simulink model "project2_model"  (R2014a)
settings: Solver=ode45  StartTime=0.0  StopTime=2  RelTol=1e-3
InitFcn:
  | G32I = [-1 -1 -1 1  1 1 -1 -1   1 1 1 1  1 -1 -1 -1   -1 1 -1 1   1 -1 -1 -1   1 1 -1 -1  -1 1 -1 1];
  | 
  | G32IR = [1 -1 1 -1 -1 -1 1 1 -1 -1 -1 1 1 -1 1 -1 -1 -1 -1 1 1 1 1 1 -1 -1 1 1  1 -1 -1 -1 ];
  | 
  | G32Q = [ 1 1 -1 1    -1 1 1 1   1 -1 1 -1   -1 1 -1 1    1 -1 1 -1   1 -1 -1 -1   -1 1 -1 1   -1 1 -1 -1  ];
  | 
  | G32QR = [ -1 -1 1 -1   1 -1 1 -1   -1 -1 -1 1   -1 1 -1 1   1 -1 1 -1   -1 1 -1 1   1  1 1 -1   1 -1 1 1 ];
libraries: simulink x3, simulink_extras x2, dspindex x2, dspsigops x1
settings Model: Creator=JohnE  LastModifiedBy=kastner

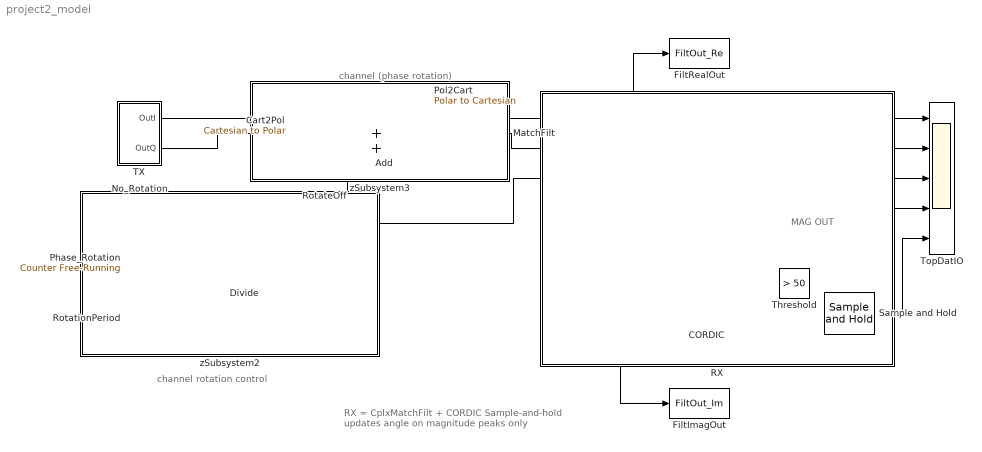
== system project2_model ==
  note: RX = CplxMatchFilt + CORDIC
      | Sample-and-hold updates angle on magnitude
      | peaks only
  note: MAG OUT
  note: channel rotation control
  note: channel (phase rotation)
  Add : Sum
  CORDIC : Subsystem
  Cart2Pol : simulink_extras/Transformations/Cartesian to Polar
  Divide : Product  Inputs=*/
  FiltImagOut : ToWorkspace  VariableName=FiltOut_Im  SaveFormat=Structure  SampleTime=-1
  FiltRealOut : ToWorkspace  VariableName=FiltOut_Re  SaveFormat=Structure  SampleTime=-1
  MatchFilt : Subsystem
  No_Rotation : Constant  Value=0
  Phase_Rotation : simulink/Sources/Counter Free-Running  NumBits=16  tsamp=-1
  Pol2Cart : simulink_extras/Transformations/Polar to Cartesian
  RX : Subsystem
      mask Display: disp('');
  RotateOff : ManualSwitch  CurrentSetting=0
  RotationPeriod : Constant  Value=1000
  Sample and Hold : dspsigops/Sample and Hold  trig=Rising edge  initCond=0  latchinput=off
  TX : Subsystem
  Threshold : simulink/Logic and Bit Operations/Compare To Constant  relop=>  const=50  OutDataTypeStr=boolean
  TopDatIO : Scope  NumInputPorts=5
      settings: YMin=-2.2~30.4~30~30.4~-5  YMax=2.2~33.6~42.5~33.6~5  SaveName=ScopeData5  MaxDataPoints=220000
  zSubsystem2 : Subsystem
      mask Display: disp('');
  zSubsystem3 : Subsystem
      mask Display: disp('');
  wires:
  MatchFilt/1(OutRe) -> CORDIC/1(XIn), TopDatIO/1, FiltRealOut/1
  MatchFilt/2(OutIm) -> FiltImagOut/1, CORDIC/2(YIn), TopDatIO/2
  TX/1(OutI) -> Cart2Pol/1
  TX/2(OutQ) -> Cart2Pol/2
  Cart2Pol/1 -> Pol2Cart/1
  Pol2Cart/1 -> MatchFilt/1(InI)
  Pol2Cart/2 -> MatchFilt/2(InQ)
  Cart2Pol/2 -> Add/1
  Add/1 -> Pol2Cart/2
  Phase_Rotation/1 -> Divide/1
  Divide/1 -> RotateOff/2
  RotationPeriod/1 -> Divide/2
  Sample and Hold/1 -> TopDatIO/5
  Threshold/1 -> Sample and Hold/Trigger
  RotateOff/1 -> Add/2, TopDatIO/3
  No_Rotation/1 -> RotateOff/1
  CORDIC/1(Mag) -> TopDatIO/4, Threshold/1
  CORDIC/2(Angle) -> Sample and Hold/1

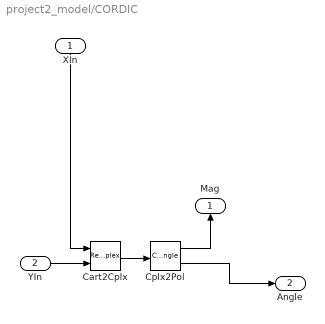
== system project2_model/CORDIC ==
  XIn : Inport
  YIn : Inport  Port=2
  Cart2Cplx : RealImagToComplex
  Cplx2Pol : ComplexToMagnitudeAngle
  Mag : Outport
  Angle : Outport  Port=2
  wires:
  XIn/1 -> Cart2Cplx/1
  YIn/1 -> Cart2Cplx/2
  Cplx2Pol/1 -> Mag/1
  Cart2Cplx/1 -> Cplx2Pol/1
  Cplx2Pol/2 -> Angle/1

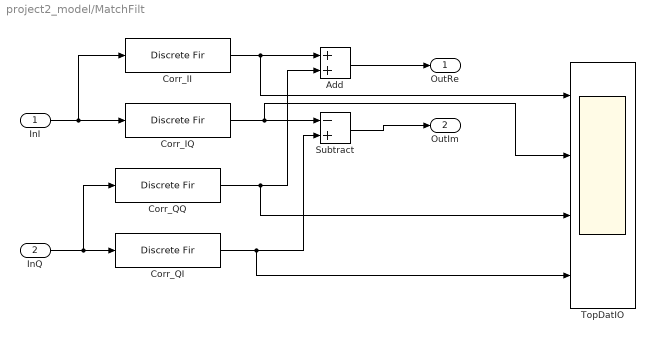
== system project2_model/MatchFilt ==
  InI : Inport
  InQ : Inport  Port=2
  Add : Sum
  Corr_II : DiscreteFir  Coefficients=G32IR
  Corr_IQ : DiscreteFir  Coefficients=G32QR
  Corr_QI : DiscreteFir  Coefficients=G32IR
  Corr_QQ : DiscreteFir  Coefficients=G32QR
  Subtract : Sum  Inputs=-+
  TopDatIO : Scope  NumInputPorts=4
      settings: YMin=-2.2~30.4~30~30.4  YMax=2.2~33.6~42.5~33.6  MaxDataPoints=220000
  OutRe : Outport
  OutIm : Outport  Port=2
  wires:
  InQ/1 -> Corr_QQ/1, Corr_QI/1
  InI/1 -> Corr_II/1, Corr_IQ/1
  Add/1 -> OutRe/1
  Corr_QQ/1 -> TopDatIO/3, Add/2
  Corr_QI/1 -> TopDatIO/4, Subtract/2
  Subtract/1 -> OutIm/1
  Corr_IQ/1 -> TopDatIO/2, Subtract/1
  Corr_II/1 -> TopDatIO/1, Add/1

== system project2_model/RX ==

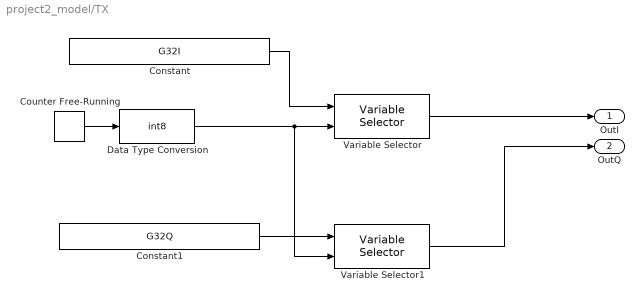
== system project2_model/TX ==
  Constant : Constant  Value=G32I  SampleTime=0.01
  Constant1 : Constant  Value=G32Q  SampleTime=0.01
  Counter Free-Running : simulink/Sources/Counter Free-Running  NumBits=5  tsamp=.01
  Data Type Conversion : DataTypeConversion  OutDataTypeStr=int8
  Variable Selector : dspindex/Variable Selector  NumInputs=1  rowsOrCols=Rows  IdxMode=Variable  Elements=[1 3]  ZerOneIdxMode=Zero-based  errmode=Clip Index  FillMode=on  FillValues=0
  Variable Selector1 : dspindex/Variable Selector  NumInputs=1  rowsOrCols=Rows  IdxMode=Variable  Elements=[1 3]  ZerOneIdxMode=Zero-based  errmode=Clip Index  FillMode=on  FillValues=0
  OutI : Outport
  OutQ : Outport  Port=2
  wires:
  Data Type Conversion/1 -> Variable Selector1/2, Variable Selector/2
  Constant1/1 -> Variable Selector1/1
  Constant/1 -> Variable Selector/1
  Variable Selector1/1 -> OutQ/1
  Variable Selector/1 -> OutI/1
  Counter Free-Running/1 -> Data Type Conversion/1

== system project2_model/zSubsystem2 ==

== system project2_model/zSubsystem3 ==
